simulink model "MymodelWired"  (R2018b)
settings: Solver=VariableStepAuto  StartTime=0.0  StopTime=10.0  RelTol=1e-3
undefined symbols (not defined in the file or in its folder): A, Ad, B, Bd, C, Cd, K_dlqr, K_kalman, Ts, x0
libraries: truetime x2
settings Model: Creator=royza  LastModifiedBy=royza

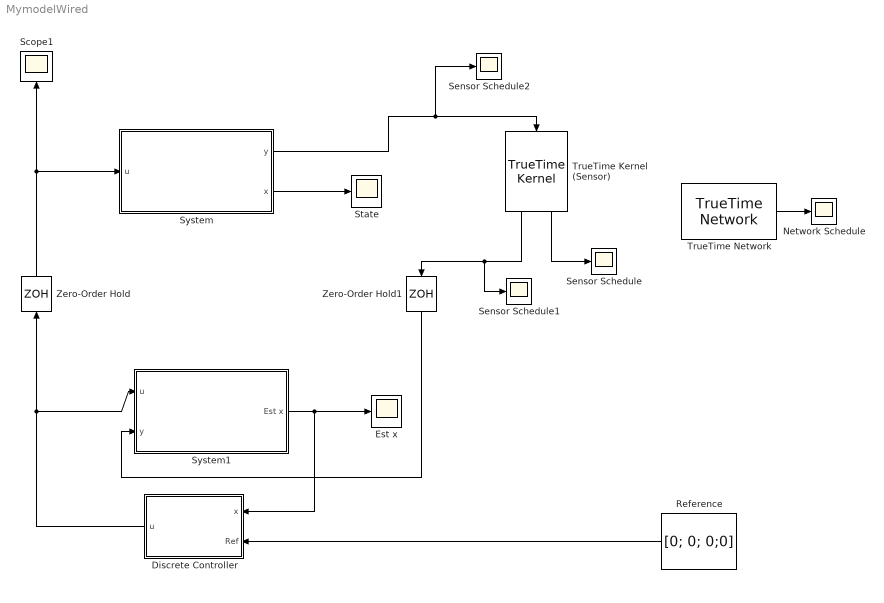
== system MymodelWired ==
  Discrete Controller : Subsystem
  Est x : Scope
  Network Schedule : Scope
  Reference : Constant  Value=[0; 0; 0;0]
  Scope1 : Scope
  Sensor Schedule : Scope
  Sensor Schedule1 : Scope
  Sensor Schedule2 : Scope
  State : Scope
  System : Subsystem
  System1 : Subsystem
  TrueTime Kernel (Sensor) : truetime/TrueTime Kernel  sfun=sensor_init  args=[]  ninputsoutputs=[1 1]  ntriggers=0  trigtype=falling  nwnodenbr=1  clockoffsetdrift=[0 0]  schedoutput=on  battery=off  poweroutput=off  label=1: 1
  TrueTime Network : truetime/TrueTime Network  nwtype=CSMA/AMP (CAN)  nwnbr=1  nnodes=1  rate=10000000  minsize=512  lossprob=0  seed=0  bandwidths=[0.5 0.5]  slotsize=512  schedule=[1 1 2]  memsize=80000  buftype=Common buffer  overflow=Retransmit  dynSchedule=0  miniSlotSize=0  NIT=0  QSortMode=FIFO  sync=0  irtSchedule=0  nrtLength=0  nodeGraph=0  scheduleoutput=on
  Zero-Order Hold : ZeroOrderHold  SampleTime=Ts
  Zero-Order Hold1 : ZeroOrderHold  SampleTime=Ts
  wires:
  System/2(x) -> State/1
  Discrete Controller/1(u) -> System1/1(u), Zero-Order Hold/1
  Reference/1 -> Discrete Controller/2(Ref)
  Zero-Order Hold/1 -> System/1(u), Scope1/1
  Zero-Order Hold1/1 -> System1/2(y)
  System1/1(Est x) -> Discrete Controller/1(x), Est x/1
  TrueTime Kernel (Sensor)/1 -> Sensor Schedule1/1, Zero-Order Hold1/1
  TrueTime Network/1 -> Network Schedule/1
  TrueTime Kernel (Sensor)/2 -> Sensor Schedule/1
  System/1(y) -> Sensor Schedule2/1, TrueTime Kernel (Sensor)/1

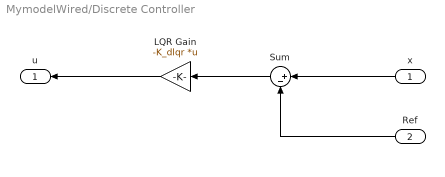
== system MymodelWired/Discrete Controller ==
  x : Inport
  Ref : Inport  Port=2
  LQR Gain : Gain  Gain=-K_dlqr  Multiplication=Matrix(K*u)
  Sum : Sum  Inputs=|+-
  u : Outport
  wires:
  LQR Gain/1 -> u/1
  x/1 -> Sum/1
  Sum/1 -> LQR Gain/1
  Ref/1 -> Sum/2

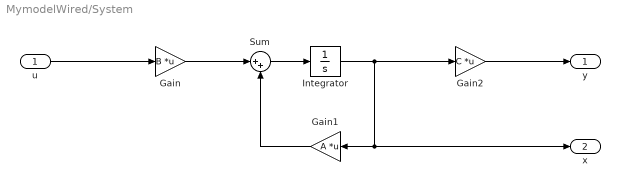
== system MymodelWired/System ==
  u : Inport
  Gain : Gain  Gain=B  Multiplication=Matrix(K*u)
  Gain1 : Gain  Gain=A  Multiplication=Matrix(K*u)
  Gain2 : Gain  Gain=C  Multiplication=Matrix(K*u)
  Integrator : Integrator  InitialCondition=x0
  Sum : Sum  Inputs=|++
  y : Outport
  x : Outport  Port=2
  wires:
  Sum/1 -> Integrator/1
  Gain/1 -> Sum/1
  Integrator/1 -> Gain2/1, x/1, Gain1/1
  Gain1/1 -> Sum/2
  u/1 -> Gain/1
  Gain2/1 -> y/1

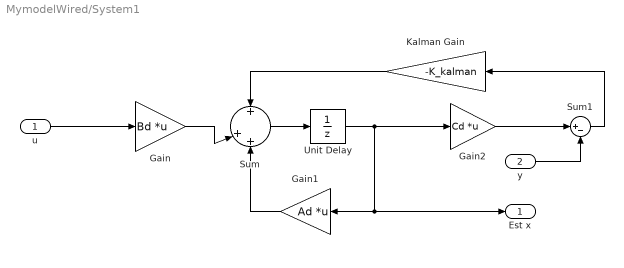
== system MymodelWired/System1 ==
  u : Inport
  y : Inport  Port=2
  Gain : Gain  Gain=Bd  Multiplication=Matrix(K*u)
  Gain1 : Gain  Gain=Ad  Multiplication=Matrix(K*u)
  Gain2 : Gain  Gain=Cd  Multiplication=Matrix(K*u)
  Kalman Gain : Gain  Gain=-K_kalman
  Sum : Sum  Inputs=+|++
  Sum1 : Sum  Inputs=|+-
  Unit Delay : UnitDelay  InitialCondition=x0*0  SampleTime=-1
  Est x : Outport
  wires:
  Gain2/1 -> Sum1/1
  u/1 -> Gain/1
  Unit Delay/1 -> Gain1/1, Est x/1, Gain2/1
  y/1 -> Sum1/2
  Sum1/1 -> Kalman Gain/1
  Sum/1 -> Unit Delay/1
  Gain1/1 -> Sum/3
  Gain/1 -> Sum/2
  Kalman Gain/1 -> Sum/1
